simulink model "GeoJacobian_Verifcation_G18"  (R2016a)
settings: Solver=VariableStepAuto  StartTime=0.0  StopTime=inf  MaxStep=1e-4  RelTol=1e-3
settings Model: Creator=Catarina  LastModifiedBy=Catarina

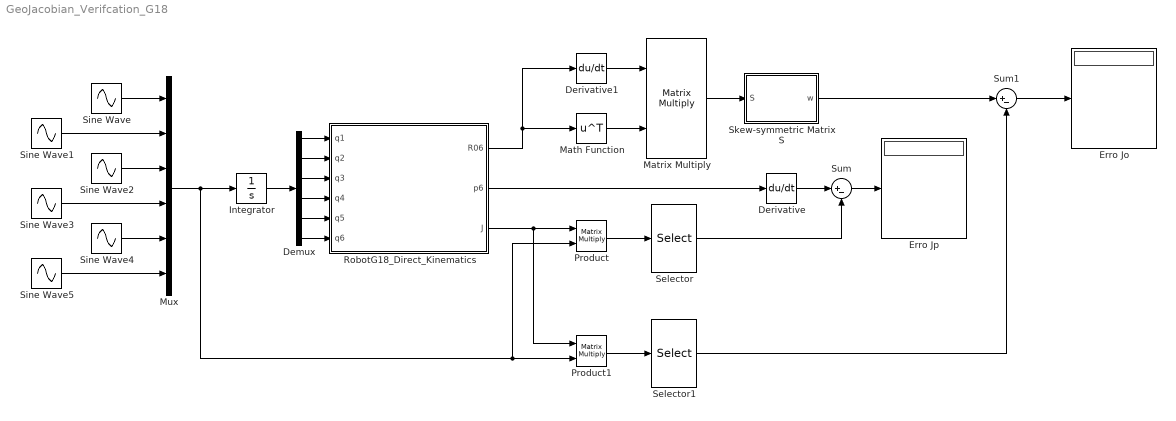
== system GeoJacobian_Verifcation_G18 ==
  Demux : Demux  Outputs=6
  Derivative : Derivative
  Derivative1 : Derivative  CoefficientInTFapproximation=0
  Erro Jo : Display
      settings: Decimation=3
  Erro Jp : Display
      settings: Decimation=3
  Integrator : Integrator
  Math Function : Math  Operator=transpose  SaturateOnIntegerOverflow=on
  Matrix Multiply : Product  Multiplication=Matrix(*)
  Mux : Mux  Inputs=6
  Product : Product  Multiplication=Matrix(*)
  Product1 : Product  Multiplication=Matrix(*)
  RobotG18_Direct_Kinematics : MATLAB Function  TreatAsAtomicUnit=on
  Selector : Selector  InputPortWidth=6  IndexOptions=Index vector (dialog)  Indices=1:3  OutputSizes=1
  Selector1 : Selector  InputPortWidth=6  IndexOptions=Index vector (dialog)  Indices=4:6  OutputSizes=1
  Sine Wave{,1..5} (6 alike) : Sin  SampleTime=0
  Skew-symmetric Matrix S : MATLAB Function  TreatAsAtomicUnit=on
  Sum : Sum  Inputs=|+-
  Sum1 : Sum  Inputs=|+-
  wires:
  Sine Wave/1 -> Mux/1
  Sine Wave1/1 -> Mux/2
  Sine Wave2/1 -> Mux/3
  Sine Wave3/1 -> Mux/4
  Sine Wave4/1 -> Mux/5
  Sine Wave5/1 -> Mux/6
  Mux/1 -> Product/2, Product1/2, Integrator/1
  Product/1 -> Selector/1
  Derivative/1 -> Sum/1
  Selector/1 -> Sum/2
  Sum/1 -> Erro Jp/1
  Integrator/1 -> Demux/1
  Demux/1 -> RobotG18_Direct_Kinematics/1(q1)
  Demux/2 -> RobotG18_Direct_Kinematics/2(q2)
  Demux/3 -> RobotG18_Direct_Kinematics/3(q3)
  Demux/4 -> RobotG18_Direct_Kinematics/4(q4)
  Demux/5 -> RobotG18_Direct_Kinematics/5(q5)
  Demux/6 -> RobotG18_Direct_Kinematics/6(q6)
  RobotG18_Direct_Kinematics/3(J) -> Product/1, Product1/1
  RobotG18_Direct_Kinematics/1(R06) -> Math Function/1, Derivative1/1
  RobotG18_Direct_Kinematics/2(p6) -> Derivative/1
  Math Function/1 -> Matrix Multiply/2
  Derivative1/1 -> Matrix Multiply/1
  Matrix Multiply/1 -> Skew-symmetric Matrix S/1(S)
  Product1/1 -> Selector1/1
  Skew-symmetric Matrix S/1(w) -> Sum1/1
  Selector1/1 -> Sum1/2
  Sum1/1 -> Erro Jo/1

== matlab function GeoJacobian_Verifcation_G18/Skew-symmetric Matrix S ==
  data: S input; w output
function w = vect(S)
%#codegen

w = [S(3,2); S(1,3); S(2,1)];

== matlab function GeoJacobian_Verifcation_G18/RobotG18_Direct_Kinematics ==
  data: q1 input; R06 output; q2 input; q3 input; q4 input; q5 input; q6 input; p6 output; J output
function [R06,p6,J] = RobotG18_Direct_Kinematics(q1,q2,q3,q4,q5,q6)
%#codegen

%    This function was generated by the Symbolic Math Toolbox version 7.0.
%    15-Apr-2021 18:49:51

t2 = q2+q3+q4;
t3 = cos(q1);
t4 = sin(q6);
t5 = sin(q1);
t6 = sin(q5);
t7 = t5.*t6;
t8 = cos(t2);
t9 = cos(q5);
t10 = t7-t3.*t8.*t9;
t11 = sin(t2);
t12 = cos(q6);
t13 = t3.*t6;
t14 = t5.*t8.*t9;
t15 = t13+t14;
t16 = q2+q3;
t17 = cos(q2);
t18 = sin(q2);
t19 = sin(q3);
t20 = cos(t16);
t21 = sin(q4);
t22 = sin(t16);
t23 = cos(q4);
t24 = cos(q3);
t25 = t5.*t17.*(1.7e1./4.0e1);
t26 = t5.*t6.*t8.*(4.1e1./5.0e2);
t27 = t5.*t17.*t24.*(4.9e1./1.25e2);
t28 = t22.*(4.9e1./1.25e2);
t29 = t18.*(1.7e1./4.0e1);
t30 = t20.*t21.*(4.1e1./5.0e2);
t31 = t22.*t23.*(4.1e1./5.0e2);
t32 = t30+t31;
t33 = t6.*t32;
t34 = t20.*t23.*(1.9e1./2.0e2);
t35 = t8.*(1.9e1./2.0e2);
t36 = t6.*t11.*(4.1e1./5.0e2);
t37 = t5.*(1.09e2./1.0e3);
t38 = t3.*t17.*(1.7e1./4.0e1);
t39 = t5.*t9.*(4.1e1./5.0e2);
t40 = t3.*t6.*t8.*(4.1e1./5.0e2);
t41 = t3.*t17.*t24.*(4.9e1./1.25e2);
t42 = t37+t38+t39+t40+t41-t3.*t18.*t19.*(4.9e1./1.25e2)-t3.*t20.*t21.*(1.9e1./2.0e2)-t3.*t22.*t23.*(1.9e1./2.0e2);
t43 = t28+t29+t33+t34-t21.*t22.*(1.9e1./2.0e2);
t44 = t28+t35+t36;
t45 = t35+t36;
t46 = q2+q3+q4+q5;
t47 = sin(t46);
t48 = t47.*(4.1e1./1.0e3);
t49 = t20.*(4.9e1./1.25e2);
t50 = q2+q3+q4-q5;
t51 = sin(t50);
t52 = t5.*t9;
t53 = t3.*t6.*t8;
t54 = t52+t53;
t55 = t5.*t6.*t8;
t56 = t55-t3.*t9;
t57 = t6.*t11;
R06 = reshape([-t10.*t12-t3.*t4.*t11,t12.*t15-t4.*t5.*t11,t4.*t8+t9.*t11.*t12,t4.*t10-t3.*t11.*t12,-t4.*t15-t5.*t11.*t12,t8.*t12-t4.*t9.*t11,t54,t56,t57],[3,3]);
if nargout > 1
    p6 = [t42;t3.*(-1.09e2./1.0e3)+t25+t26+t27-t3.*t9.*(4.1e1./5.0e2)-t5.*t18.*t19.*(4.9e1./1.25e2)-t5.*t20.*t21.*(1.9e1./2.0e2)-t5.*t22.*t23.*(1.9e1./2.0e2);t28+t29+t33+t34-t21.*t22.*(1.9e1./2.0e2)+8.9e1./1.0e3];
end
if nargout > 2
    J = reshape([t3.*(1.09e2./1.0e3)-t25-t26-t27+t3.*t9.*(4.1e1./5.0e2)+t5.*t18.*t19.*(4.9e1./1.25e2)+t5.*t20.*t21.*(1.9e1./2.0e2)+t5.*t22.*t23.*(1.9e1./2.0e2),t42,0.0,0.0,0.0,1.0,-t3.*t43,-t5.*t43,t11.*(-1.9e1./2.0e2)+t17.*(1.7e1./4.0e1)+t48+t49-t51.*(4.1e1./1.0e3),t5,-t3,0.0,-t3.*t44,-t5.*t44,t11.*(-1.9e1./2.0e2)+t48+t49-t51.*(4.1e1./1.0e3),t5,-t3,0.0,-t3.*t45,-t5.*t45,t11.*(-1.9e1./2.0e2)+t48-t51.*(4.1e1./1.0e3),t5,-t3,0.0,t5.*t6.*(-4.1e1./5.0e2)-t3.*t9.*t17.*t19.*t21.*(4.1e1./5.0e2)-t3.*t9.*t18.*t19.*t23.*(4.1e1./5.0e2)-t3.*t9.*t18.*t21.*t24.*(4.1e1./5.0e2)+t3.*t9.*t17.*t23.*t24.*(4.1e1./5.0e2),t3.*t6.*(4.1e1./5.0e2)-t5.*t9.*t17.*t19.*t21.*(4.1e1./5.0e2)-t5.*t9.*t18.*t19.*t23.*(4.1e1./5.0e2)-t5.*t9.*t18.*t21.*t24.*(4.1e1./5.0e2)+t5.*t9.*t17.*t23.*t24.*(4.1e1./5.0e2),t48+t51.*(4.1e1./1.0e3),-t3.*t11,-t5.*t11,t8,0.0,0.0,0.0,t54,t56,t57],[6,6]);
end
